simulink model "mogen_SMU_test"  (Simulink 9.2)
settings: Solver=ode4  StartTime=0.0  StopTime=6  FixedStep=model_sample_time  RelTol=1e-3
undefined symbols (not defined in the file): magnitude, model_sample_time
libraries: utils x4, simulink x2
(part 1 of 3)
settings Model: Creator=msrm  LastModifiedBy=msrm  SnapshotBufferSize=100  SnapshotInterval=1
settings DataIOCC: ExternalInput=ds  LimitDataPoints=off  SaveFormat=Dataset  SignalLoggingSaveFormat=Dataset  SaveOutput=off  SignalLogging=off  DSMLogging=off  SaveTime=off
settings OptimizationCC: OptimizeBlockIOStorage=off  BufferReuse=off  GlobalBufferReuse=off  ExpressionFolding=off  LocalBlockOutputs=off  LifeSpan=auto  OptimizeDataStoreBuffers=off  BusAssignmentInplaceUpdate=off
settings DebuggingCC: UnderspecifiedInitializationDetection=Simplified  MergeDetectMultiDrivingBlocksExec=error  FcnCallInpInsideContextMsg=error  StateNameClashWarn=none  SFUnexpectedBacktrackingDiag=error  SFNoUnconditionalDefaultTransitionDiag=error  SFExecutionAtInitializationDiag=warning
settings HardwareCC: ProdBitPerPointer=64  ProdBitPerSizeT=64  ProdBitPerPtrDiffT=64  ProdLargestAtomicFloat=Float  ProdIntDivRoundTo=Zero  ProdEndianess=LittleEndian  ProdWordSize=64  ProdHWDeviceType=Intel->x86-64 (Windows64)
settings ModelReferenceCC: PropagateSignalLabelsOutOfModel=on
settings SFSimCC: SimUseLocalCustomCode=on
settings RTWCC: GenCodeOnly=on  RTWUseLocalCustomCode=on  BuildConfiguration=Debug  TargetLang=C++  RTWCompilerOptimization=Custom  RTWCustomCompilerOptimizations=O3  CheckMdlBeforeBuild=Warning
settings CodeAppCC: ForceParamTrailComments=on  StateflowObjectComments=off  MATLABSourceComments=on
settings GRTTargetCC: TargetLangStandard=C++03 (ISO)  GeneratePreprocessorConditionals=Use local settings  CombineOutputUpdateFcns=on  MultiInstanceERTCode=on  CodeInterfacePackaging=C++ class  GRTInterface=off  MultiInstanceErrorCode=Warning
settings CPPComponent: GenerateDestructor=on  GenerateExternalIOAccessMethods=None  ParameterMemberVisibility=private  InternalMemberVisibility=private  GenerateParameterAccessMethods=None  GenerateInternalMemberAccessMethods=None  UseOperatorNewForModelRefRegistration=off
settings ConfigComp: CovMetricSettings=dwe  CovHtmlReporting=off  CovSaveCumulativeToWorkspaceVar=off  CovSaveSingleToWorkspaceVar=off  CovExternalEMLEnable=on

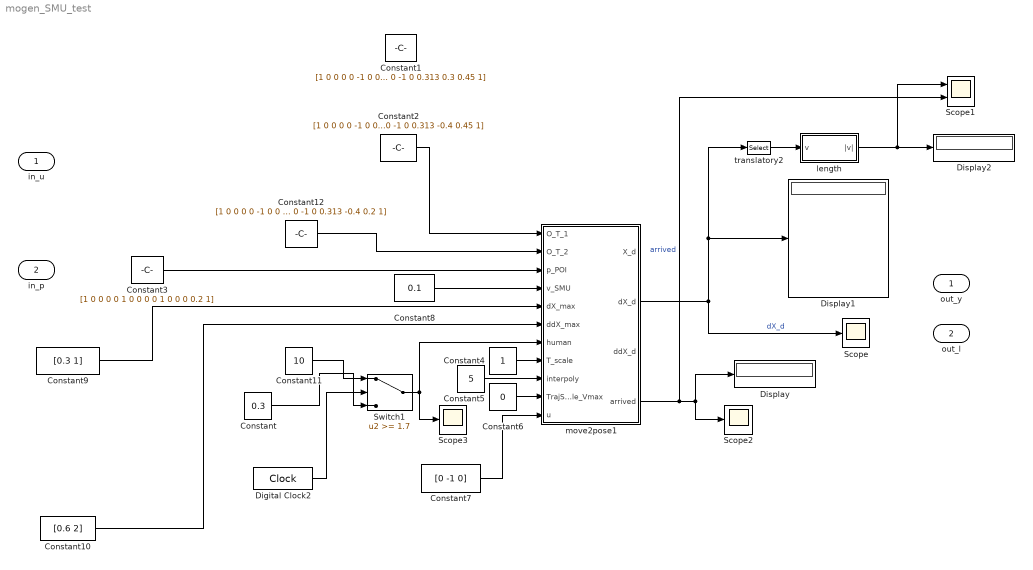
== system mogen_SMU_test ==
  in_u : Inport  OutDataTypeStr=Bus: in_u
  in_p : Inport  Port=2  OutDataTypeStr=Bus: in_p
  Constant : Constant  Value=0.3
  Constant1 : Constant  Value=[1 0 0 0 0 -1 0 0 0 0 -1 0 0.313 0.3 0.45 1]
  Constant10 : Constant  Value=[0.6 2]
  Constant11 : Constant  Value=10
  Constant12 : Constant  Value=[1 0 0 0 0 -1 0 0 0 0 -1 0 0.313 -0.4 0.2 1]
  Constant2 : Constant  Value=[1 0 0 0 0 -1 0 0 0 0 -1 0 0.313 -0.4 0.45 1]  VectorParams1D=off
  Constant3 : Constant  Value=[1 0 0 0 0 1 0 0 0 0 1 0 0 0 0.2 1]
  Constant4 : Constant
  Constant5 : Constant  Value=5
  Constant6 : Constant  Value=0
  Constant7 : Constant  Value=[0 -1 0]
  Constant8 : Constant  Value=0.1
  Constant9 : Constant  Value=[0.3 1]
  Digital Clock2 : DigitalClock  SampleTime=model_sample_time
  Display : Display
  Display1 : Display
  Display2 : Display
  Scope : Scope
  Scope1 : Scope  NumInputPorts=2
  Scope2 : Scope
  Scope3 : Scope
  Switch1 : Switch  Threshold=1.7
  length : Subsystem
  move2pose1 : Subsystem
  translatory2 : Selector  InputPortWidth=6  IndexOptions=Index vector (dialog)  Indices=[1:3]  OutputSizes=1
  out_y : Outport  OutDataTypeStr=Bus: out_y
  out_l : Outport  Port=2  OutDataTypeStr=Bus: out_l
  wires:
  move2pose1/2(dX_d) -> translatory2/1, Display1/1, Scope/1  "dX_d"
  Constant12/1 -> move2pose1/2(O_T_2)
  Constant2/1 -> move2pose1/1(O_T_1)
  Constant3/1 -> move2pose1/3(p_POI)
  Constant4/1 -> move2pose1/8(T_scale)
  Constant5/1 -> move2pose1/9(interpoly)
  Constant6/1 -> move2pose1/10(TrajScale_Vmax)
  Constant7/1 -> move2pose1/11(u)
  Constant8/1 -> move2pose1/4(v_SMU)
  Constant9/1 -> move2pose1/5(dX_max)
  Constant10/1 -> move2pose1/6(ddX_max)
  move2pose1/4(arrived) -> Scope1/2, Display/1, Scope2/1  "arrived"
  translatory2/1 -> length/1(v)
  length/1(|v|) -> Scope1/1, Display2/1
  Constant/1 -> Switch1/1
  Constant11/1 -> Switch1/3
  Switch1/1 -> move2pose1/7(human), Scope3/1
  Digital Clock2/1 -> Switch1/2

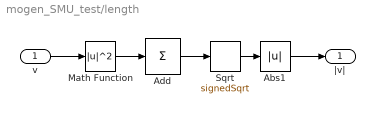
== system mogen_SMU_test/length ==
  v : Inport
  Abs1 : Abs
  Add : Sum  Inputs=+
  Math Function : Math  Operator=magnitude^2  SaturateOnIntegerOverflow=on
  Sqrt : Sqrt  Operator=signedSqrt  SaturateOnIntegerOverflow=on
  |v| : Outport
  wires:
  Math Function/1 -> Add/1
  Add/1 -> Sqrt/1
  v/1 -> Math Function/1
  Abs1/1 -> |v|/1
  Sqrt/1 -> Abs1/1

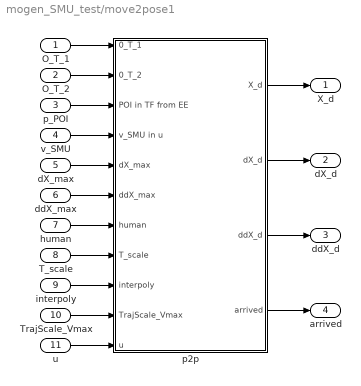
== system mogen_SMU_test/move2pose1 ==
  O_T_1 : Inport
  O_T_2 : Inport  Port=2
  p_POI : Inport  Port=3
  v_SMU : Inport  Port=4
  dX_max : Inport  Port=5
  ddX_max : Inport  Port=6
  human : Inport  Port=7
  T_scale : Inport  Port=8
  interpoly : Inport  Port=9
  TrajScale_Vmax : Inport  Port=10
  u : Inport  Port=11
  p2p : Subsystem
  X_d : Outport
  dX_d : Outport  Port=2
  ddX_d : Outport  Port=3
  arrived : Outport  Port=4
  wires:
  p2p/4(arrived) -> arrived/1
  dX_max/1 -> p2p/5(dX_max)
  p2p/2(dX_d) -> dX_d/1
  ddX_max/1 -> p2p/6(ddX_max)
  O_T_1/1 -> p2p/1(0_T_1)
  O_T_2/1 -> p2p/2(0_T_2)
  human/1 -> p2p/7(human)
  T_scale/1 -> p2p/8(T_scale)
  interpoly/1 -> p2p/9(interpoly)
  TrajScale_Vmax/1 -> p2p/10(TrajScale_Vmax)
  p_POI/1 -> p2p/3(POI in TF from EE)
  u/1 -> p2p/11(u)
  v_SMU/1 -> p2p/4(v_SMU in u)
  p2p/1(X_d) -> X_d/1
  p2p/3(ddX_d) -> ddX_d/1

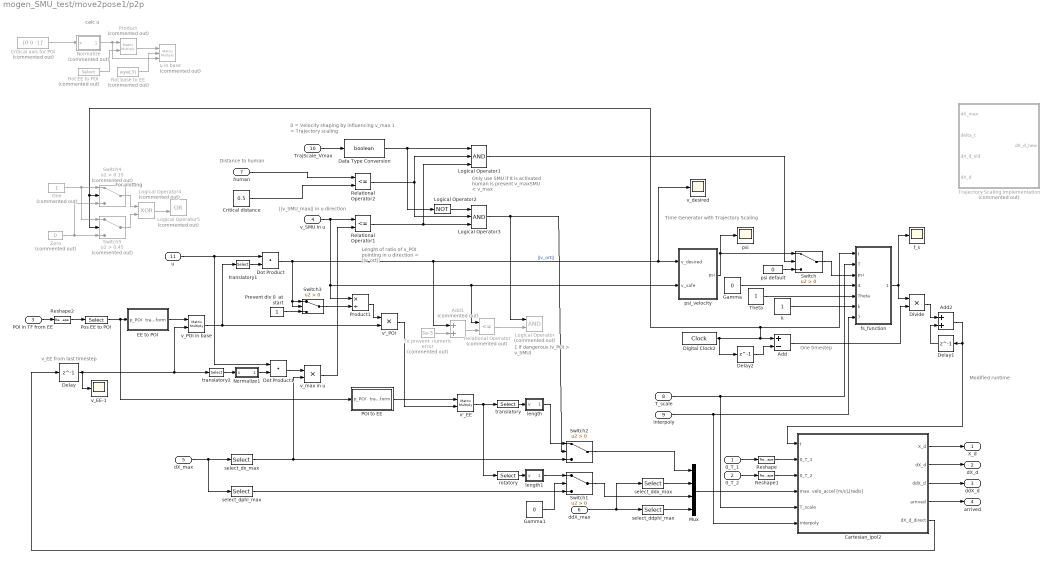
== system mogen_SMU_test/move2pose1/p2p ==
  note: calc u
  note: Distance to human
  note: For plotting
  note: v_EE from last timestep
  note: ||v_SMU_max|| in u direction
  note: Modified runtime
  note: One timestep
  note: Only use SMU if
      | It is activated
      | human is present
      | v_maxSMU < v_max
  note: 0 = Velocity shaping by influencing v_max
      | 1 = Trajectory scaling
  note: 1 if dangerous
      | (v_POI > v_SMU)
  note: Lenght of ratio of v_POI
      | pointing in u direction
      | = ||v_ort||
  note: Time Generator with Trajectory Scaling
  0_T_1 : Inport
  0_T_2 : Inport  Port=2
  POI in TF from EE : Inport  Port=3
  v_SMU in u : Inport  Port=4
  dX_max : Inport  Port=5
  ddX_max : Inport  Port=6
  human : Inport  Port=7
  T_scale : Inport  Port=8
  interpoly : Inport  Port=9
  TrajScale_Vmax : Inport  Port=10
  u : Inport  Port=11
  Add : Sum  Inputs=+-
  Add1 : Sum  Commented=on
  Add2 : Sum
  Cartesian_ipol2 : Subsystem  TreatAsAtomicUnit=on
  Critical axis for POI : Constant  Commented=on  Value=[0 0 -1]'
  Critical distance : Constant  Value=0.5
  Data Type Conversion : DataTypeConversion  OutDataTypeStr=boolean
  Delay : Delay  DelayLength=1
  Delay1 : Delay  DelayLength=1
  Delay2 : Delay  DelayLength=1
  Digital Clock2 : DigitalClock  SampleTime=model_sample_time
  Divide : Product  Inputs=**
  Dot Product : DotProduct  InputSameDT=on  OutDataTypeStr=Inherit: Inherit via internal rule
  Dot Product1 : DotProduct  InputSameDT=on  OutDataTypeStr=Inherit: Inherit via internal rule
  EE to POI : MATLAB Function  TreatAsAtomicUnit=on
  Gamma : Constant  Value=0
  Gamma1 : Constant  Value=0
  Logical Operator : Logic  Commented=on  AllPortsSameDT=off  OutDataTypeStr=boolean
  Logical Operator1 : Logic  Inputs=3  AllPortsSameDT=off  OutDataTypeStr=boolean
  Logical Operator2 : Logic  Operator=NOT  AllPortsSameDT=off  OutDataTypeStr=boolean
  Logical Operator3 : Logic  Inputs=3  AllPortsSameDT=off  OutDataTypeStr=boolean
  Logical Operator4 : Logic  Commented=on  Operator=XOR  AllPortsSameDT=off  OutDataTypeStr=boolean
  Logical Operator5 : Logic  Commented=on  Operator=OR  AllPortsSameDT=off  OutDataTypeStr=boolean
  Mux : Mux
  Normalize : Subsystem  Commented=on
  Normalize1 : Subsystem
  One : Constant  Commented=on
  POI to EE : MATLAB Function  TreatAsAtomicUnit=on
  Pos EE to POI : Selector  NumberOfDimensions=2  InputPortWidth=7  IndexOptions=Index vector (dialog),Index vector (dialog)  Indices=[1:3],[4]  OutputSizes=1
  Prevent div 0  at start : Constant
  Product : Product  Commented=on  Multiplication=Matrix(*)
  Product1 : Product  Inputs=*/
  Relational Operator : RelationalOperator  Commented=on  Operator=<=  OutDataTypeStr=boolean  RndMeth=Simplest
  Relational Operator1 : RelationalOperator  Operator=<=  OutDataTypeStr=boolean  RndMeth=Simplest
  Relational Operator2 : RelationalOperator  Operator=<=  OutDataTypeStr=boolean  RndMeth=Simplest
  Reshape : Reshape  OutputDimensionality=Customize  OutputDimensions=[4,4]
  Reshape1 : Reshape  OutputDimensionality=Customize  OutputDimensions=[4,4]
  Reshape2 : Reshape  OutputDimensionality=Customize  OutputDimensions=[4,4]
  Rot EE to POI : Selector  Commented=on  NumberOfDimensions=2  InputPortWidth=7  IndexOptions=Index vector (dialog),Index vector (dialog)  Indices=[1:3],[1:3]  OutputSizes=1
  Rot base to EE : Constant  Commented=on  Value=eye(3)
  Switch{,1..3} (4 alike) : Switch  Criteria=u2 > Threshold
  Switch4 : Switch  Commented=on  Criteria=u2 > Threshold  Threshold=0.15
  Switch5 : Switch  Commented=on  Criteria=u2 > Threshold  Threshold=0.45
  Theta : Constant
  To prevent  numeric error : Constant  Commented=on  Value=3e-3
  Trajectory Scaling Implementation : MATLAB Function  Commented=on  TreatAsAtomicUnit=on
  Zero : Constant  Commented=on  Value=0
  f_s : Scope
  fs_function : MATLAB Function  TreatAsAtomicUnit=on
  k : Constant
  length : Subsystem
  length1 : Subsystem
  psi : Scope
  psi default : Constant  Value=0
  psi_velocity : MATLAB Function  TreatAsAtomicUnit=on
  rotatory : Selector  InputPortWidth=6  IndexOptions=Index vector (dialog)  Indices=[4:6]  OutputSizes=1
  select_ddphi_max : Selector  InputPortWidth=2  IndexOptions=Index vector (dialog)  Indices=2  OutputSizes=1
  select_ddx_max : Selector  InputPortWidth=2  IndexOptions=Index vector (dialog)  Indices=1  OutputSizes=1
  select_dphi_max : Selector  InputPortWidth=2  IndexOptions=Index vector (dialog)  Indices=2  OutputSizes=1
  select_dx_max : Selector  InputPortWidth=2  IndexOptions=Index vector (dialog)  Indices=1  OutputSizes=1
  translatory : Selector  InputPortWidth=6  IndexOptions=Index vector (dialog)  Indices=[1:3]  OutputSizes=1
  translatory1 : Selector  InputPortWidth=6  IndexOptions=Index vector (dialog)  Indices=[1:3]  OutputSizes=1
  translatory2 : Selector  InputPortWidth=6  IndexOptions=Index vector (dialog)  Indices=[1:3]  OutputSizes=1
  u in base : Product  Commented=on  Inputs=3  Multiplication=Matrix(*)
  v'_EE : Product  Multiplication=Matrix(*)
  v'_POI : Product
  v_EE-1 : Scope
  v_POI in base : Product  Multiplication=Matrix(*)
  v_desired : Scope
  v_max in u : Product
  X_d : Outport
  dX_d : Outport  Port=2
  ddX_d : Outport  Port=3
  arrived : Outport  Port=4
  wires:
  0_T_2/1 -> Reshape1/1
  0_T_1/1 -> Reshape/1
  ddX_max/1 -> select_ddx_max/1, select_ddphi_max/1
  select_ddphi_max/1 -> Mux/4
  Mux/1 -> Cartesian_ipol2/4(max. velo_accel [m/s],[rad/s])
  select_dphi_max/1 -> Switch1/3
  select_ddx_max/1 -> Mux/2
  Digital Clock2/1 -> Delay2/1, Switch4/2, Switch5/2, fs_function/1(t), Add/1
  Delay2/1 -> Add/2
  Divide/1 -> Add2/1
  Delay1/1 -> Add2/2
  Cartesian_ipol2/4(arrived) -> arrived/1
  Gamma/1 -> fs_function/4(Gamma)
  k/1 -> fs_function/6(k)
  Theta/1 -> fs_function/5(Theta)
  Cartesian_ipol2/2(dX_d) -> dX_d/1
  psi_velocity/1(psi) -> psi/1, Switch/1
  Critical axis for POI/1 -> Normalize/1(x)
  Normalize/1(x/||x||) -> u in base/3, Product/1
  dX_max/1 -> select_dphi_max/1, select_dx_max/1
  TrajScale_Vmax/1 -> Data Type Conversion/1
  Data Type Conversion/1 -> Logical Operator1/1, Logical Operator2/1
  Logical Operator2/1 -> Logical Operator3/1
  Switch2/1 -> Mux/1
  v_SMU in u/1 -> Product1/1, psi_velocity/2(v_safe), Relational Operator/1, Relational Operator1/1
  Add/1 -> Divide/2
  Relational Operator2/1 -> Logical Operator3/2, Logical Operator1/2
  Dot Product/1 -> v_desired/1, psi_velocity/1(v_desired), Add1/1, Switch3/2, Switch3/1  "||v_ort||"
  interpoly/1 -> Cartesian_ipol2/6(interpoly), fs_function/7(interpoly)
  T_scale/1 -> fs_function/2(T), Cartesian_ipol2/5(T_scale)
  fs_function/1(time_factor) -> Divide/1, f_s/1
  psi default/1 -> Switch/3
  Logical Operator1/1 -> Switch/2
  Switch/1 -> fs_function/3(psi)
  Add2/1 -> Delay1/1, Cartesian_ipol2/1(t)
  Cartesian_ipol2/5(dX_d_direct) -> Delay/1
  Rot EE to POI/1 -> Product/2
  POI in TF from EE/1 -> Reshape2/1
  Product/1 -> u in base/1
  Rot base to EE/1 -> u in base/2
  EE to POI/1(transform) -> v_POI in base/1
  Delay/1 -> v_POI in base/2, translatory2/1, v_EE-1/1
  v_POI in base/1 -> v'_POI/2, translatory1/1
  Product1/1 -> v'_POI/1
  length/1(|v|) -> Switch2/1
  v'_POI/1 -> v'_EE/2
  POI to EE/1(transform) -> v'_EE/1
  v'_EE/1 -> translatory/1, rotatory/1
  translatory/1 -> length/1(v)
  Relational Operator1/1 -> Logical Operator1/3, Logical Operator3/3
  translatory1/1 -> Dot Product/2
  Pos EE to POI/1 -> POI to EE/1(p_POI), EE to POI/1(p_POI)
  Switch1/1 -> Mux/3
  rotatory/1 -> length1/1(v)
  length1/1(|v|) -> Switch1/1
  translatory2/1 -> Normalize1/1(x)
  Normalize1/1(x/||x||) -> Dot Product1/2
  Dot Product1/1 -> v_max in u/1
  v_max in u/1 -> Relational Operator1/2
  To prevent  numeric error/1 -> Add1/2
  Add1/1 -> Relational Operator/2
  select_dx_max/1 -> v_max in u/2, Switch2/3
  Switch4/1 -> Logical Operator4/1
  Switch5/1 -> Logical Operator4/2
  Zero/1 -> Switch5/3, Switch4/3
  One/1 -> Switch4/1, Switch5/1
  human/1 -> Relational Operator2/1
  Critical distance/1 -> Relational Operator2/2
  u/1 -> Dot Product/1, Dot Product1/1
  Switch3/1 -> Product1/2
  Prevent div 0  at start/1 -> Switch3/3
  Logical Operator4/1 -> Logical Operator5/2
  Cartesian_ipol2/3(ddX_d) -> ddX_d/1
  Cartesian_ipol2/1(X_d) -> X_d/1
  Reshape/1 -> Cartesian_ipol2/2(0_T_1)
  Reshape1/1 -> Cartesian_ipol2/3(0_T_2)
  Reshape2/1 -> Pos EE to POI/1
  Relational Operator/1 -> Logical Operator/2
  Gamma1/1 -> Switch1/2
  Logical Operator3/1 -> Switch2/2, Logical Operator/1

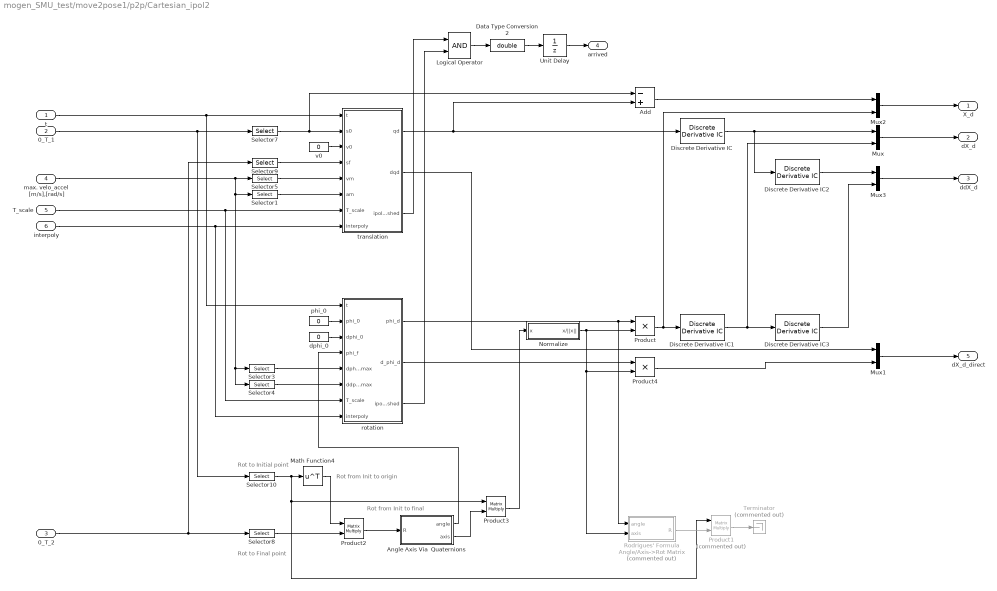
== system mogen_SMU_test/move2pose1/p2p/Cartesian_ipol2 ==
  note: Rot from
      | Init to final
  note: Rot from Init to origin
  note: Rot to Initial point
  note: Rot to Final point
  t : Inport
  0_T_1 : Inport  Port=2
  0_T_2 : Inport  Port=3
  max. velo_accel [m/s],[rad/s] : Inport  Port=4
  T_scale : Inport  Port=5
  interpoly : Inport  Port=6
  Add : Sum  Inputs=-+
  Angle Axis Via  Quaternions : Subsystem
  Data Type Conversion2 : DataTypeConversion  OutDataTypeStr=double
  Discrete Derivative IC{,1..3} (4 alike) : utils/Discrete Derivative IC  model_sample_time=model_sample_time
  Logical Operator : Logic  AllPortsSameDT=off  OutDataTypeStr=boolean
  Math Function4 : Math  Operator=transpose  SaturateOnIntegerOverflow=on
  Mux{,1..3} (4 alike) : Mux  Inputs=2
  Normalize : Subsystem
  Product : Product
  Product1 : Product  Commented=on  Multiplication=Matrix(*)  RndMeth=Zero
  Product2 : Product  Multiplication=Matrix(*)  RndMeth=Zero
  Product3 : Product  Multiplication=Matrix(*)
  Product4 : Product
  "Rodrigues' Formula Angle/Axis->Rot Matrix " : Subsystem  Commented=on
  Selector1 : Selector  InputPortWidth=4  IndexOptions=Index vector (dialog)  Indices=2  OutputSizes=1
  Selector10 : Selector  NumberOfDimensions=2  InputPortWidth=7  IndexOptions=Index vector (dialog),Index vector (dialog)  Indices=[1:3],[1:3]  OutputSizes=1
  Selector3 : Selector  InputPortWidth=4  IndexOptions=Index vector (dialog)  Indices=3  OutputSizes=1
  Selector4 : Selector  InputPortWidth=4  IndexOptions=Index vector (dialog)  Indices=4  OutputSizes=1
  Selector5 : Selector  InputPortWidth=4  IndexOptions=Index vector (dialog)  Indices=1  OutputSizes=1
  Selector7 : Selector  NumberOfDimensions=2  InputPortWidth=7  IndexOptions=Index vector (dialog),Index vector (dialog)  Indices=[1:3],[4]  OutputSizes=1
  Selector8 : Selector  NumberOfDimensions=2  InputPortWidth=7  IndexOptions=Index vector (dialog),Index vector (dialog)  Indices=[1:3],[1:3]  OutputSizes=1
  Selector9 : Selector  NumberOfDimensions=2  InputPortWidth=7  IndexOptions=Index vector (dialog),Index vector (dialog)  Indices=[1:3],[4]  OutputSizes=1
  Terminator : Terminator  Commented=on
  Unit Delay : UnitDelay  SampleTime=-1
  dphi_0 : Constant  Value=0
  phi_0 : Constant  Value=0
  rotation : Subsystem
  translation : Subsystem
  v0 : Constant  Value=0
  X_d : Outport
  dX_d : Outport  Port=2
  ddX_d : Outport  Port=3
  arrived : Outport  Port=4
  dX_d_direct : Outport  Port=5
  wires:
  0_T_1/1 -> Selector10/1, Selector7/1
  Selector1/1 -> translation/6(am)
  max. velo_accel [m/s],[rad/s]/1 -> Selector4/1, Selector3/1, Selector1/1, Selector5/1
  Data Type Conversion2/1 -> Unit Delay/1
  dphi_0/1 -> rotation/3(dphi_0)
  Selector10/1 -> Product3/1, Product1/1, Math Function4/1
  Angle Axis Via  Quaternions/1(angle) -> rotation/4(phi_f)
  Product2/1 -> Angle Axis Via  Quaternions/1(R)
  Selector8/1 -> Product2/2
  Math Function4/1 -> Product2/1
  Selector9/1 -> translation/4(sf)
  Selector3/1 -> rotation/5(dphi_max)
  Selector4/1 -> rotation/6(ddphi_max)
  rotation/1(phi_d) -> "Rodrigues' Formula Angle/Axis->Rot Matrix "/1(angle), Product/1
  "Rodrigues' Formula Angle/Axis->Rot Matrix "/1(R) -> Product1/2
  phi_0/1 -> rotation/2(phi_0)
  Selector7/1 -> Add/1, translation/2(s0)
  Selector5/1 -> translation/5(vm)
  v0/1 -> translation/3(v0)
  Normalize/1(x/||x||) -> Product4/2, "Rodrigues' Formula Angle/Axis->Rot Matrix "/2(axis), Product/2
  0_T_2/1 -> Selector9/1, Selector8/1
  Mux/1 -> dX_d/1
  Product1/1 -> Terminator/1
  Angle Axis Via  Quaternions/2(axis) -> Product3/2
  Product3/1 -> Normalize/1(x)
  t/1 -> rotation/1(t), translation/1(t)
  Product/1 -> Mux2/2, Discrete Derivative IC1/1
  translation/1(qd) -> Discrete Derivative IC/1, Add/2
  T_scale/1 -> rotation/7(T_scale), translation/7(T_scale)
  interpoly/1 -> translation/8(interpoly), rotation/8(interpoly)
  Discrete Derivative IC/1 -> Discrete Derivative IC2/1, Mux/1
  translation/2(dqd) -> Mux1/1
  Mux1/1 -> dX_d_direct/1
  rotation/2(d_phi_d) -> Product4/1
  Product4/1 -> Mux1/2
  Unit Delay/1 -> arrived/1
  translation/3(ipol_finished) -> Logical Operator/1
  Logical Operator/1 -> Data Type Conversion2/1
  Mux2/1 -> X_d/1
  Add/1 -> Mux2/1
  Mux3/1 -> ddX_d/1
  Discrete Derivative IC2/1 -> Mux3/1
  Discrete Derivative IC3/1 -> Mux3/2
  Discrete Derivative IC1/1 -> Mux/2, Discrete Derivative IC3/1
  rotation/3(ipol_finished) -> Logical Operator/2

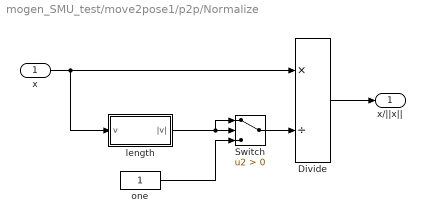
== system mogen_SMU_test/move2pose1/p2p/Normalize ==
  x : Inport
  Divide : Product  Inputs=*/
  Switch : Switch  Criteria=u2 > Threshold
  length : Subsystem
  one : Constant
  x/||x|| : Outport
  wires:
  x/1 -> Divide/1, length/1(v)
  Divide/1 -> x/||x||/1
  one/1 -> Switch/3
  length/1(|v|) -> Switch/2, Switch/1
  Switch/1 -> Divide/2

== system mogen_SMU_test/move2pose1/p2p/Normalize1 ==
  x : Inport
  Divide : Product  Inputs=*/
  Switch : Switch  Criteria=u2 > Threshold
  length : Subsystem
  one : Constant
  x/||x|| : Outport
  wires:
  x/1 -> Divide/1, length/1(v)
  Divide/1 -> x/||x||/1
  one/1 -> Switch/3
  length/1(|v|) -> Switch/2, Switch/1
  Switch/1 -> Divide/2

== system mogen_SMU_test/move2pose1/p2p/length ==
  v : Inport
  Abs1 : Abs
  Add : Sum  Inputs=+
  Math Function : Math  Operator=magnitude^2  SaturateOnIntegerOverflow=on
  Sqrt : Sqrt  Operator=signedSqrt  SaturateOnIntegerOverflow=on
  |v| : Outport
  wires:
  Math Function/1 -> Add/1
  Add/1 -> Sqrt/1
  v/1 -> Math Function/1
  Abs1/1 -> |v|/1
  Sqrt/1 -> Abs1/1

== system mogen_SMU_test/move2pose1/p2p/length1 ==
  v : Inport
  Abs1 : Abs
  Add : Sum  Inputs=+
  Math Function : Math  Operator=magnitude^2  SaturateOnIntegerOverflow=on
  Sqrt : Sqrt  Operator=signedSqrt  SaturateOnIntegerOverflow=on
  |v| : Outport
  wires:
  Math Function/1 -> Add/1
  Add/1 -> Sqrt/1
  v/1 -> Math Function/1
  Abs1/1 -> |v|/1
  Sqrt/1 -> Abs1/1

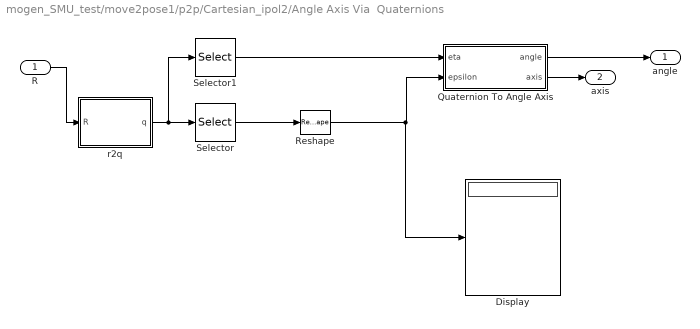
== system mogen_SMU_test/move2pose1/p2p/Cartesian_ipol2/Angle Axis Via  Quaternions ==
  R : Inport
  Display : Display
  Quaternion To Angle Axis : Subsystem
  Reshape : Reshape  OutputDimensionality=Column vector (2-D)
  Selector : Selector  InputPortWidth=4  IndexOptions=Index vector (dialog)  Indices=2:4  OutputSizes=1
  Selector1 : Selector  InputPortWidth=4  IndexOptions=Index vector (dialog)  Indices=1  OutputSizes=1
  r2q : MATLAB Function  TreatAsAtomicUnit=on
  angle : Outport
  axis : Outport  Port=2
  wires:
  Quaternion To Angle Axis/2(axis) -> axis/1
  R/1 -> r2q/1(R)
  Quaternion To Angle Axis/1(angle) -> angle/1
  Selector/1 -> Reshape/1
  Selector1/1 -> Quaternion To Angle Axis/1(eta)
  r2q/1(q) -> Selector1/1, Selector/1
  Reshape/1 -> Display/1, Quaternion To Angle Axis/2(epsilon)

== system mogen_SMU_test/move2pose1/p2p/Cartesian_ipol2/Normalize ==
  x : Inport
  Divide : Product  Inputs=*/
  Switch : Switch  Criteria=u2 > Threshold
  length : Subsystem
  one : Constant
  x/||x|| : Outport
  wires:
  x/1 -> Divide/1, length/1(v)
  Divide/1 -> x/||x||/1
  one/1 -> Switch/3
  length/1(|v|) -> Switch/2, Switch/1
  Switch/1 -> Divide/2

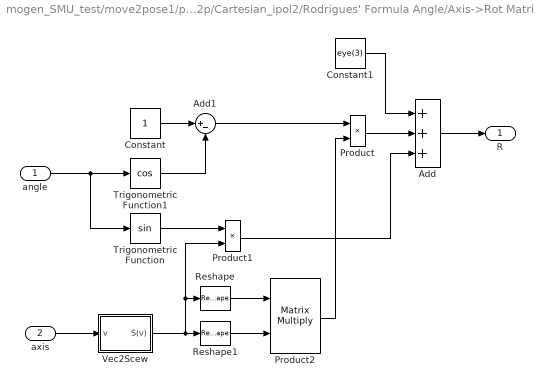
== system mogen_SMU_test/move2pose1/p2p/Cartesian_ipol2/Rodrigues' Formula Angle/Axis->Rot Matrix  ==
  angle : Inport
  axis : Inport  Port=2
  Add : Sum  Inputs=+++
  Add1 : Sum  Inputs=|+-
  Constant : Constant
  Constant1 : Constant  Value=eye(3)
  Product : Product  RndMeth=Zero
  Product1 : Product  RndMeth=Zero
  Product2 : Product  Multiplication=Matrix(*)  RndMeth=Zero
  Reshape : Reshape  OutputDimensionality=Customize  OutputDimensions=[3,3]
  Reshape1 : Reshape  OutputDimensionality=Customize  OutputDimensions=[3,3]
  Trigonometric Function : Trigonometry
  Trigonometric Function1 : Trigonometry  Operator=cos
  Vec2Scew : Subsystem
      mask help:
      | Converts a 3-vector to a scew symmetric matrix accroding to the 'tilde'-operator,
      | i.e. S(v)=[0, -v(3), v(2); v(3), 0, -v(1); -v(2), v(1), 0].
  R : Outport
  wires:
  Reshape1/1 -> Product2/2
  Reshape/1 -> Product2/1
  Product2/1 -> Product/2
  Constant1/1 -> Add/1
  Product/1 -> Add/2
  Product1/1 -> Add/3
  Vec2Scew/1(S(v)) -> Reshape1/1, Reshape/1, Product1/2
  Trigonometric Function/1 -> Product1/1
  Add1/1 -> Product/1
  Trigonometric Function1/1 -> Add1/2
  Constant/1 -> Add1/1
  Add/1 -> R/1
  angle/1 -> Trigonometric Function1/1, Trigonometric Function/1
  axis/1 -> Vec2Scew/1(v)

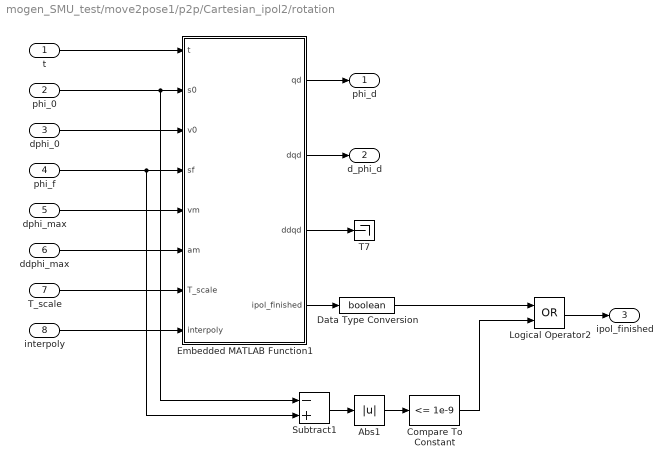
== system mogen_SMU_test/move2pose1/p2p/Cartesian_ipol2/rotation ==
  t : Inport
  phi_0 : Inport  Port=2
  dphi_0 : Inport  Port=3
  phi_f : Inport  Port=4
  dphi_max : Inport  Port=5
  ddphi_max : Inport  Port=6
  T_scale : Inport  Port=7
  interpoly : Inport  Port=8
  Abs1 : Abs
  Compare To Constant : simulink/Logic and Bit Operations/Compare To Constant  relop=<=  const=1e-9  OutDataTypeStr=boolean
  Data Type Conversion : DataTypeConversion  OutDataTypeStr=boolean
  Embedded MATLAB Function1 : MATLAB Function  TreatAsAtomicUnit=on
  Logical Operator2 : Logic  Operator=OR  AllPortsSameDT=off  OutDataTypeStr=boolean
  Subtract1 : Sum  Inputs=-+
  T7 : Terminator
  phi_d : Outport
  d_phi_d : Outport  Port=2
  ipol_finished : Outport  Port=3
  wires:
  ddphi_max/1 -> Embedded MATLAB Function1/6(am)
  dphi_max/1 -> Embedded MATLAB Function1/5(vm)
  phi_f/1 -> Subtract1/2, Embedded MATLAB Function1/4(sf)
  dphi_0/1 -> Embedded MATLAB Function1/3(v0)
  phi_0/1 -> Subtract1/1, Embedded MATLAB Function1/2(s0)
  Embedded MATLAB Function1/1(qd) -> phi_d/1
  t/1 -> Embedded MATLAB Function1/1(t)
  Embedded MATLAB Function1/3(ddqd) -> T7/1
  Embedded MATLAB Function1/2(dqd) -> d_phi_d/1
  interpoly/1 -> Embedded MATLAB Function1/8(interpoly)
  T_scale/1 -> Embedded MATLAB Function1/7(T_scale)
  Compare To Constant/1 -> Logical Operator2/2
  Subtract1/1 -> Abs1/1
  Abs1/1 -> Compare To Constant/1
  Logical Operator2/1 -> ipol_finished/1
  Embedded MATLAB Function1/4(ipol_finished) -> Data Type Conversion/1
  Data Type Conversion/1 -> Logical Operator2/1

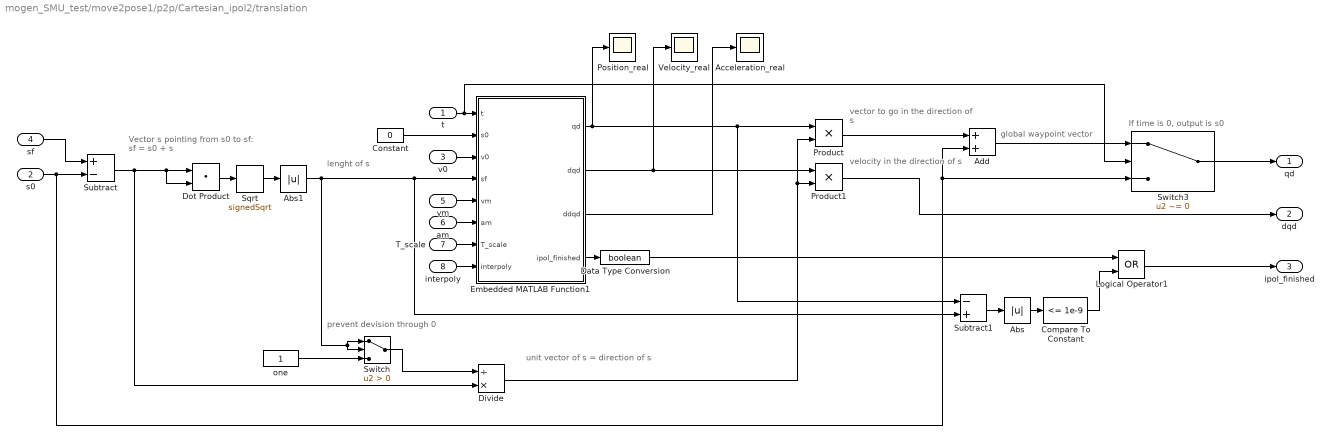
== system mogen_SMU_test/move2pose1/p2p/Cartesian_ipol2/translation ==
  note: vector to go in
      | the direction of s
  note: unit vector of s
      | = direction of s
  note: lenght of s
  note: Vector s pointing
      | from s0 to sf:
      |  sf = s0 + s
  note: global waypoint vector
  note: If time is 0, output is s0
  note: prevent devision
      | through 0
  note: velocity in
      | the direction of s
  t : Inport
  s0 : Inport  Port=2
  v0 : Inport  Port=3
  sf : Inport  Port=4
  vm : Inport  Port=5
  am : Inport  Port=6
  T_scale : Inport  Port=7
  interpoly : Inport  Port=8
  Abs : Abs
  Abs1 : Abs
  Acceleration_real : Scope
  Add : Sum
  Compare To Constant : simulink/Logic and Bit Operations/Compare To Constant  relop=<=  const=1e-9  OutDataTypeStr=boolean
  Constant : Constant  Value=0
  Data Type Conversion : DataTypeConversion  OutDataTypeStr=boolean
  Divide : Product  Inputs=/*
  Dot Product : DotProduct  OutMin=0  InputSameDT=on  OutDataTypeStr=Inherit: Inherit via internal rule
  Embedded MATLAB Function1 : MATLAB Function  TreatAsAtomicUnit=on
  Logical Operator1 : Logic  Operator=OR  AllPortsSameDT=off  OutDataTypeStr=boolean
  Position_real : Scope
  Product : Product
  Product1 : Product
  Sqrt : Sqrt  Operator=signedSqrt  SaturateOnIntegerOverflow=on
  Subtract : Sum  Inputs=+-
  Subtract1 : Sum  Inputs=-+
  Switch : Switch  Criteria=u2 > Threshold
  Switch3 : Switch  Criteria=u2 ~= 0
  Velocity_real : Scope
  one : Constant
  qd : Outport
  dqd : Outport  Port=2
  ipol_finished : Outport  Port=3
  wires:
  Switch3/1 -> qd/1
  Logical Operator1/1 -> ipol_finished/1
  Embedded MATLAB Function1/2(dqd) -> Product1/1, Velocity_real/1
  Embedded MATLAB Function1/1(qd) -> Product/1, Subtract1/1, Position_real/1
  Sqrt/1 -> Abs1/1
  Constant/1 -> Embedded MATLAB Function1/2(s0)
  t/1 -> Switch3/2, Embedded MATLAB Function1/1(t)
  am/1 -> Embedded MATLAB Function1/6(am)
  vm/1 -> Embedded MATLAB Function1/5(vm)
  v0/1 -> Embedded MATLAB Function1/3(v0)
  s0/1 -> Add/2, Switch3/3, Subtract/2
  sf/1 -> Subtract/1
  Subtract/1 -> Dot Product/2, Dot Product/1, Divide/2
  Dot Product/1 -> Sqrt/1
  Divide/1 -> Product1/2, Product/2
  Product/1 -> Add/1
  Add/1 -> Switch3/1
  Subtract1/1 -> Abs/1
  Compare To Constant/1 -> Logical Operator1/2
  Abs/1 -> Compare To Constant/1
  one/1 -> Switch/3
  Switch/1 -> Divide/1
  Embedded MATLAB Function1/3(ddqd) -> Acceleration_real/1
  T_scale/1 -> Embedded MATLAB Function1/7(T_scale)
  interpoly/1 -> Embedded MATLAB Function1/8(interpoly)
  Product1/1 -> dqd/1
  Abs1/1 -> Subtract1/2, Embedded MATLAB Function1/4(sf), Switch/1, Switch/2
  Embedded MATLAB Function1/4(ipol_finished) -> Data Type Conversion/1
  Data Type Conversion/1 -> Logical Operator1/1

== system mogen_SMU_test/move2pose1/p2p/Normalize/length ==
  v : Inport
  Add : Sum  Inputs=+
  Math Function : Math  Operator=magnitude^2  SaturateOnIntegerOverflow=on
  Math Function1 : Math  Operator=sqrt  SaturateOnIntegerOverflow=on
  |v| : Outport
  wires:
  Math Function/1 -> Add/1
  Add/1 -> Math Function1/1
  v/1 -> Math Function/1
  Math Function1/1 -> |v|/1

== system mogen_SMU_test/move2pose1/p2p/Normalize1/length ==
  v : Inport
  Abs1 : Abs
  Add : Sum  Inputs=+
  Math Function : Math  Operator=magnitude^2  SaturateOnIntegerOverflow=on
  Sqrt : Sqrt  Operator=signedSqrt  SaturateOnIntegerOverflow=on
  |v| : Outport
  wires:
  Math Function/1 -> Add/1
  Add/1 -> Sqrt/1
  v/1 -> Math Function/1
  Abs1/1 -> |v|/1
  Sqrt/1 -> Abs1/1

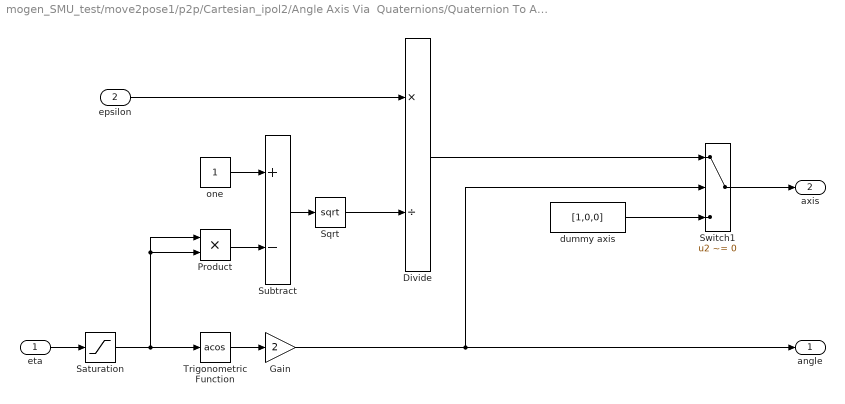
== system mogen_SMU_test/move2pose1/p2p/Cartesian_ipol2/Angle Axis Via  Quaternions/Quaternion To Angle Axis ==
  eta : Inport
  epsilon : Inport  Port=2
  Divide : Product  Inputs=*/
  Gain : Gain  Gain=2
  Product : Product  RndMeth=Zero
  Saturation : Saturate  UpperLimit=1  LowerLimit=-1
  Sqrt : Sqrt  SaturateOnIntegerOverflow=on
  Subtract : Sum  Inputs=+-
  Switch1 : Switch  Criteria=u2 ~= 0
  Trigonometric Function : Trigonometry  Operator=acos
  dummy axis : Constant  Value=[1,0,0]
  one : Constant
  angle : Outport
  axis : Outport  Port=2
  wires:
  Divide/1 -> Switch1/1
  Switch1/1 -> axis/1
  dummy axis/1 -> Switch1/3
  Gain/1 -> Switch1/2, angle/1
  epsilon/1 -> Divide/1
  Trigonometric Function/1 -> Gain/1
  eta/1 -> Saturation/1
  Subtract/1 -> Sqrt/1
  one/1 -> Subtract/1
  Product/1 -> Subtract/2
  Sqrt/1 -> Divide/2
  Saturation/1 -> Trigonometric Function/1, Product/1, Product/2

== system mogen_SMU_test/move2pose1/p2p/Cartesian_ipol2/Normalize/length ==
  v : Inport
  Abs1 : Abs
  Add : Sum  Inputs=+
  Math Function : Math  Operator=magnitude^2  SaturateOnIntegerOverflow=on
  Sqrt : Sqrt  Operator=signedSqrt  SaturateOnIntegerOverflow=on
  |v| : Outport
  wires:
  Math Function/1 -> Add/1
  Add/1 -> Sqrt/1
  v/1 -> Math Function/1
  Abs1/1 -> |v|/1
  Sqrt/1 -> Abs1/1

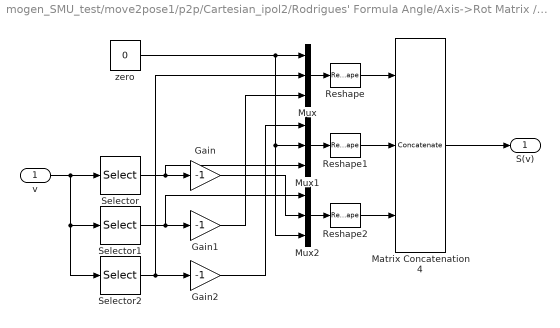
== system mogen_SMU_test/move2pose1/p2p/Cartesian_ipol2/Rodrigues' Formula Angle/Axis->Rot Matrix /Vec2Scew ==
  v : Inport
  Gain : Gain  Gain=-1  SaturateOnIntegerOverflow=on  OutDataTypeStr=Inherit: Same as input  ParamDataTypeStr=Inherit: Same as input
  Gain1 : Gain  Gain=-1  SaturateOnIntegerOverflow=on  OutDataTypeStr=Inherit: Same as input  ParamDataTypeStr=Inherit: Same as input
  Gain2 : Gain  Gain=-1  SaturateOnIntegerOverflow=on  OutDataTypeStr=Inherit: Same as input  ParamDataTypeStr=Inherit: Same as input
  Matrix Concatenation4 : Concatenate  NumInputs=3  Mode=Multidimensional array  ConcatenateDimension=2
  Mux : Mux  Inputs=3
  Mux1 : Mux  Inputs=3
  Mux2 : Mux  Inputs=3
  Reshape : Reshape  OutputDimensionality=Customize  OutputDimensions=[3,1]
  Reshape1 : Reshape  OutputDimensionality=Customize  OutputDimensions=[3,1]
  Reshape2 : Reshape  OutputDimensionality=Customize  OutputDimensions=[3,1]
  Selector : Selector  InputPortWidth=3  IndexOptions=Index vector (dialog)  Indices=[1]  OutputSizes=1
  Selector1 : Selector  InputPortWidth=3  IndexOptions=Index vector (dialog)  Indices=[2]  OutputSizes=1
  Selector2 : Selector  InputPortWidth=3  IndexOptions=Index vector (dialog)  Indices=[3]  OutputSizes=1
  zero : Constant  Value=0
  S(v) : Outport
  wires:
  zero/1 -> Mux1/2, Mux2/3, Mux/1
  Selector/1 -> Gain/1, Mux1/3
  Selector1/1 -> Gain1/1, Mux2/1
  Selector2/1 -> Gain2/1, Mux/2
  Gain1/1 -> Mux/3
  Gain2/1 -> Mux1/1
  Gain/1 -> Mux2/2
  v/1 -> Selector/1, Selector1/1, Selector2/1
  Matrix Concatenation4/1 -> S(v)/1
  Reshape1/1 -> Matrix Concatenation4/2
  Mux2/1 -> Reshape2/1
  Mux/1 -> Reshape/1
  Reshape/1 -> Matrix Concatenation4/1
  Mux1/1 -> Reshape1/1
  Reshape2/1 -> Matrix Concatenation4/3

== matlab function move2pose1/p2p/Cartesian_ipol2/Angle Axis Via Quaternions/r2q ==
  data: R input double; q output double
function q =r2q(R)
%#codegen
q=zeros(1,4);
if ~(all(size(R)==[3,3]))
    error('Bad input dimensions. Input must be 3x3');
end

% Ne dela za specialne kote, ko je s=0 ali v=0
% s=0.5*sqrt(R(1,1)+R(2,2)+R(3,3)+1);
% v=[R(3,2)-R(2,3),R(1,3)-R(3,1),R(2,1)-R(1,2)]'/4/s;
%
% q=quaternion([s v']);

qsx=trace(R)+1;
if qsx>=0
    qs = sqrt(qsx)/2.0;
else
    qs=0;
end
kx = R(3,2) - R(2,3);	% Oz - Ay
ky = R(1,3) - R(3,1);	% Ax - Nz
kz = R(2,1) - R(1,2);	% Ny - Ox

if (R(1,1) >= R(2,2)) && (R(1,1) >= R(3,3))
    kx1 = R(1,1) - R(2,2) - R(3,3) + 1;	% Nx - Oy - Az + 1
    ky1 = R(2,1) + R(1,2);			% Ny + Ox
    kz1 = R(3,1) + R(1,3);			% Nz + Ax
    add = (kx >= 0);
elseif (R(2,2) >= R(3,3))
    kx1 = R(2,1) + R(1,2);			% Ny + Ox
    ky1 = R(2,2) - R(1,1) - R(3,3) + 1;	% Oy - Nx - Az + 1
    kz1 = R(3,2) + R(2,3);			% Oz + Ay
    add = (ky >= 0);
else
    kx1 = R(3,1) + R(1,3);			% Nz + Ax
    ky1 = R(3,2) + R(2,3);			% Oz + Ay
    kz1 = R(3,3) - R(1,1) - R(2,2) + 1;	% Az - Nx - Oy + 1
    add = (kz >= 0);
end

if add
    kx = kx + kx1;
    ky = ky + ky1;
    kz = kz + kz1;
else
    kx = kx - kx1;
    ky = ky - ky1;
    kz = kz - kz1;
end
nm = norm([kx ky kz]);
if nm == 0
    q = [1 0 0 0];
else
    ss=1-qs^2;
    if ss<0
        s=0;
    else
        s = sqrt(ss) / nm;
    end
    qv = s*[kx ky kz];
    
    q = [qs qv];
end
